simulink subsystem "FirstHouse"  (R2023a)
settings: Solver=VariableStepAuto  StartTime=0.0  StopTime=10.0  RelTol=1e-3
undefined symbols (not defined in the file): A
libraries: mpclib x1
settings Model: Creator=giaco  LastModifiedBy=giaco

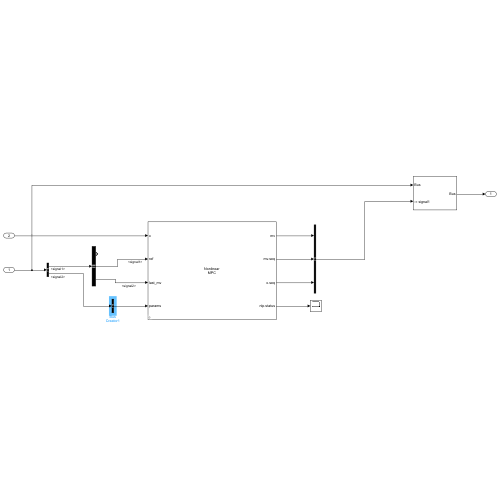
[thumbnail: Simulink's stored preview of the top-level diagram]
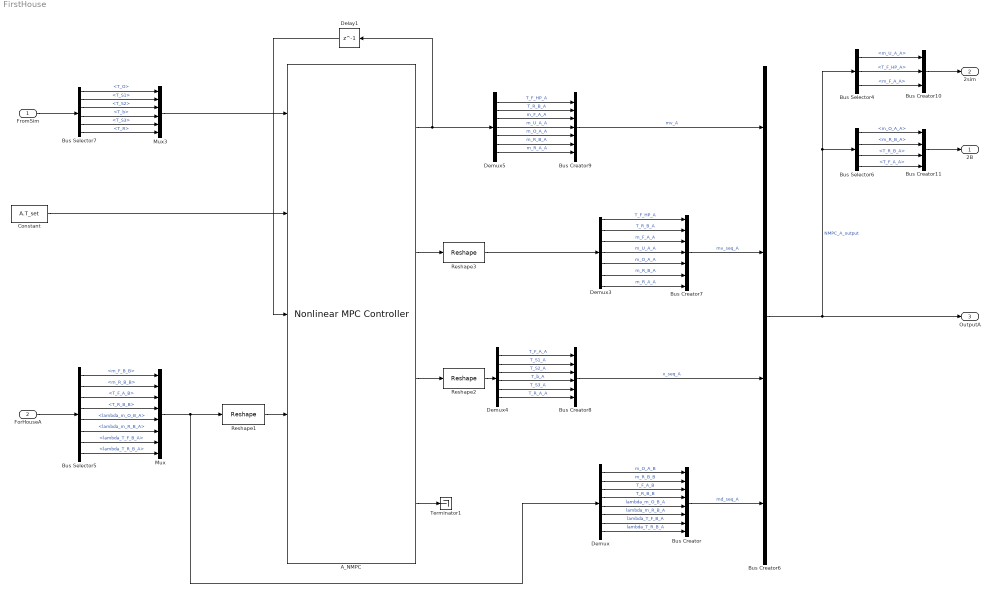
== system FirstHouse ==
  FromSim : Inport
  ForHouseA : Inport  Port=2
  A_NMPC : mpclib/Nonlinear MPC Controller  nlmpcobj=A.nlobj  UseObjectTs=on  UseMEX=off  md_enabled=on  mvtarget_enabled=off  param_enabled=on  cost_enabled=off  mvseq_enabled=on  stateseq_enabled=on  ovseq_enabled=off  slack_enabled=off  status_enabled=on  ov_min=off  ov_max=off  mv_min=off  mv_max=off  mvrate_min=off  mvrate_max=off  state_min=off  state_max=off  ov_weight=off  mv_weight=off  mvrate_weight=off  ecr_weight=off  nlp_initialize=off
  Bus Creator : BusCreator  Inputs=8  OutDataTypeStr=Bus: Bus_md_seq_A
  Bus Creator10 : BusCreator  Inputs=3
  Bus Creator11 : BusCreator  Inputs=4
  Bus Creator6 : BusCreator  Inputs=4  OutDataTypeStr=Bus: NMPC_A_output
  Bus Creator7 : BusCreator  Inputs=7  OutDataTypeStr=Bus: Bus_mv_seq_A
  Bus Creator8 : BusCreator  Inputs=6  OutDataTypeStr=Bus: Bus_x_seq_A
  Bus Creator9 : BusCreator  Inputs=7  OutDataTypeStr=Bus: Bus_mv_A
  Bus Selector4 : BusSelector  OutputSignals=mv_A.m_U_A_A,mv_A.T_F_HP_A,mv_A.m_F_A_A
  Bus Selector5 : BusSelector  OutputSignals=B2A.m_F_B_B,B2A.m_R_B_B,B2A.T_F_A_B,B2A.T_R_B_B,A_storage.md_seq.lambda_m_O_B_A,A_storage.md_seq.lambda_m_R_B_A,A_storage.md_seq.lambda_T_F_B_A,A_storage.md_seq.lambda_T_R_B_A
  Bus Selector6 : BusSelector  OutputSignals=mv_seq_A.m_O_A_A,mv_seq_A.m_R_B_A,mv_seq_A.T_R_B_A,x_seq_A.T_F_A_A
  Bus Selector7 : BusSelector  OutputSignals=T_O,T_S1,T_S2,T_b,T_S3,T_R
  Constant : Constant  Value=A.T_set
  Delay1 : Delay  DelayLength=1
  Demux : Demux  Outputs=8
  Demux3 : Demux  Outputs=7
  Demux4 : Demux  Outputs=6
  Demux5 : Demux  Outputs=7
  Mux : Mux  Inputs=8
  Mux3 : Mux  Inputs=6
  Reshape1 : Reshape  OutputDimensionality=Customize  OutputDimensions=[A.K, A.nu_md]
  Reshape2 : Reshape  OutputDimensionality=Customize  OutputDimensions=[(A.K+1) * A.nx, 1]
  Reshape3 : Reshape  OutputDimensionality=Customize  OutputDimensions=[(A.K+1) * A.nu_mv, 1]
  Terminator1 : Terminator
  2B : Outport
  2sim : Outport  Port=2
  OutputA : Outport  Port=3
  wires:
  Demux4/2 -> Bus Creator8/2  "T_S1_A"
  Bus Selector6/2 -> Bus Creator11/2  "<m_R_B_A>"
  Bus Creator6/1 -> OutputA/1, Bus Selector6/1, Bus Selector4/1  "NMPC_A_output"
  Demux4/4 -> Bus Creator8/4  "T_b_A"
  A_NMPC/4 -> Terminator1/1
  Mux3/1 -> A_NMPC/1
  Demux5/1 -> Bus Creator9/1  "T_F_HP_A"
  Bus Selector4/1 -> Bus Creator10/1  "<m_U_A_A>"
  Bus Selector6/3 -> Bus Creator11/3  "<T_R_B_A>"
  Demux5/4 -> Bus Creator9/4  "m_U_A_A"
  Demux4/5 -> Bus Creator8/5  "T_S3_A"
  Bus Selector6/1 -> Bus Creator11/1  "<m_O_A_A>"
  Bus Selector6/4 -> Bus Creator11/4  "<T_F_A_A>"
  Demux4/3 -> Bus Creator8/3  "T_S2_A"
  Demux4/6 -> Bus Creator8/6  "T_R_A_A"
  Bus Creator11/1 -> 2B/1
  Bus Selector4/2 -> Bus Creator10/2  "<T_F_HP_A>"
  Demux4/1 -> Bus Creator8/1  "T_F_A_A"
  Reshape1/1 -> A_NMPC/4
  Bus Creator10/1 -> 2sim/1
  Demux5/5 -> Bus Creator9/5  "m_O_A_A"
  Bus Creator8/1 -> Bus Creator6/3  "x_seq_A"
  Demux5/7 -> Bus Creator9/7  "m_R_A_A"
  Demux5/3 -> Bus Creator9/3  "m_F_A_A"
  Demux5/2 -> Bus Creator9/2  "T_R_B_A"
  Bus Selector4/3 -> Bus Creator10/3  "<m_F_A_A>"
  Bus Creator7/1 -> Bus Creator6/2  "mv_seq_A"
  A_NMPC/3 -> Reshape2/1
  Mux/1 -> Reshape1/1, Demux/1
  FromSim/1 -> Bus Selector7/1
  Delay1/1 -> A_NMPC/3
  Bus Creator9/1 -> Bus Creator6/1  "mv_A"
  Demux5/6 -> Bus Creator9/6  "m_R_B_A"
  Demux3/6 -> Bus Creator7/6  "m_R_B_A"
  Demux3/2 -> Bus Creator7/2  "T_R_B_A"
  Demux3/3 -> Bus Creator7/3  "m_F_A_A"
  Demux3/7 -> Bus Creator7/7  "m_R_A_A"
  Demux3/5 -> Bus Creator7/5  "m_O_A_A"
  Demux3/1 -> Bus Creator7/1  "T_F_HP_A"
  Demux3/4 -> Bus Creator7/4  "m_U_A_A"
  A_NMPC/2 -> Reshape3/1
  Bus Selector7/1 -> Mux3/1  "<T_O>"
  Bus Selector7/2 -> Mux3/2  "<T_S1>"
  Bus Selector7/3 -> Mux3/3  "<T_S2>"
  Bus Selector7/4 -> Mux3/4  "<T_b>"
  Bus Selector7/5 -> Mux3/5  "<T_S3>"
  Bus Selector7/6 -> Mux3/6  "<T_R>"
  Constant/1 -> A_NMPC/2
  ? -> A_NMPC/5
  Demux/5 -> Bus Creator/5  "lambda_m_O_B_A"
  Demux/7 -> Bus Creator/7  "lambda_T_F_B_A"
  Demux/8 -> Bus Creator/8  "lambda_T_R_B_A"
  Demux/4 -> Bus Creator/4  "T_R_B_B"
  Demux/6 -> Bus Creator/6  "lambda_m_R_B_A"
  Demux/2 -> Bus Creator/2  "m_R_B_B"
  Demux/1 -> Bus Creator/1  "m_O_A_B"
  Demux/3 -> Bus Creator/3  "T_F_A_B"
  Bus Selector5/1 -> Mux/1  "<m_F_B_B>"
  Bus Selector5/2 -> Mux/2  "<m_R_B_B>"
  Bus Selector5/3 -> Mux/3  "<T_F_A_B>"
  Bus Selector5/4 -> Mux/4  "<T_R_B_B>"
  Bus Creator/1 -> Bus Creator6/4  "md_seq_A"
  Bus Selector5/8 -> Mux/8  "<lambda_T_R_B_A>"
  Bus Selector5/5 -> Mux/5  "<lambda_m_O_B_A>"
  Bus Selector5/6 -> Mux/6  "<lambda_m_R_B_A>"
  Bus Selector5/7 -> Mux/7  "<lambda_T_F_B_A>"
  ForHouseA/1 -> Bus Selector5/1
  Reshape2/1 -> Demux4/1
  Reshape3/1 -> Demux3/1
  A_NMPC/1 -> Delay1/1, Demux5/1
